simulink model "task2"  (R2025b)
settings: Solver=VariableStepAuto  StartTime=0.0  StopTime=24  RelTol=1e-3
values from neighbouring files (symbols this model uses):
  Pf = 1.5    [init.m]
  Pr = 7.0    (= 7)    [init.m]
  Sb_0 = 0.55    [init.m]
  Ta_0 = 10.0    (= 10)    [init.m]
  Tp_0 = 11.5    [init.m]
libraries: slpidlib x2
settings Model: Creator=davide  LastModifiedBy=davide

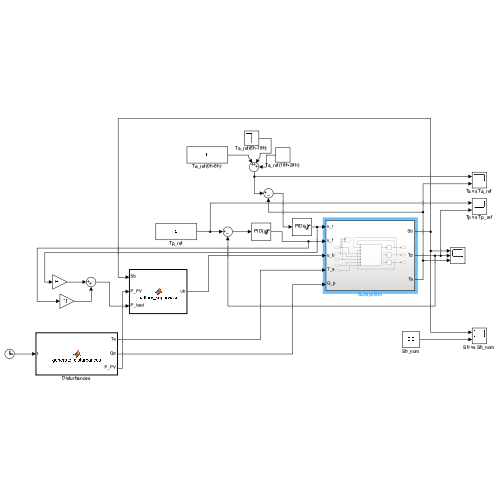
[thumbnail: Simulink's stored preview of the top-level diagram]
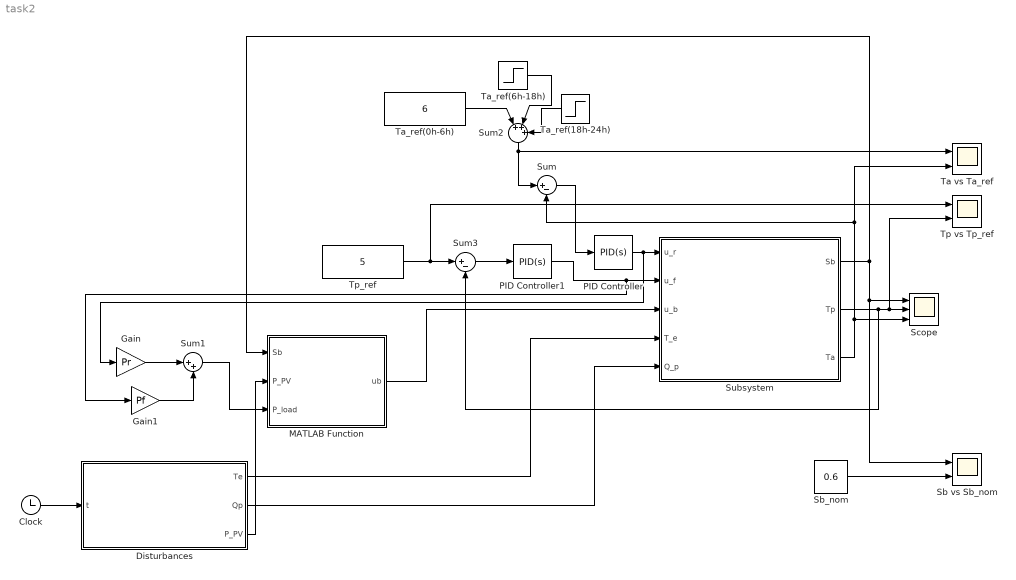
== system task2 ==
  Clock : Clock
  Disturbances : MATLAB Function  TreatAsAtomicUnit=on
  Gain : Gain  Gain=Pr
  Gain1 : Gain  Gain=Pf
  MATLAB Function : MATLAB Function  TreatAsAtomicUnit=on
  PID Controller : slpidlib/PID Controller  Controller=PID  Form=Parallel  TimeDomain=Continuous-time  UseExternalTs=off  SampleTime=-1  IntegratorMethod=Forward Euler  FilterMethod=Forward Euler  ControllerParametersSource=internal  P=-0.5  I=-1  UseKiTs=off  D=0  UseExternalDerivativeSource=off  N=100  UseFilter=on  TunerSelectOption=Transfer Function Based (PID Tuner App)  InitialConditionSource=internal  InitialConditionForIntegrator=0  InitialConditionForFilter=0  DifferentiatorICPrevScaledInput=0  ExternalReset=none  TrackingMode=off  Kt=1  LimitOutput=on  SatLimitsSource=internal  UpperSaturationLimit=1  LowerSaturationLimit=0  LinearizeAsGain=on  AntiWindupMode=back-calculation  Kb=1  LimitIntegrator=off  UpperIntegratorSaturationLimit=inf  LowerIntegratorSaturationLimit=-inf  POutMin=[]  POutMax=[]  IOutMin=[]  IOutMax=[]  DOutMin=[]  DOutMax=[]  NOutMin=[]  NOutMax=[]  SumOutMin=[]  SumOutMax=[]  SaturationOutMin=[]  SaturationOutMax=[]  PParamMin=[]  PParamMax=[]  IParamMin=[]  IParamMax=[]  DParamMin=[]  DParamMax=[]  NParamMin=[]  NParamMax=[]  KbParamMin=[]  KbParamMax=[]  KtParamMin=[]  KtParamMax=[]  KbOutMin=[]  KbOutMax=[]  KtOutMin=[]  KtOutMax=[]  IntegratorOutMin=[]  IntegratorOutMax=[]  FilterOutMin=[]  FilterOutMax=[]  SumI1OutMin=[]  SumI1OutMax=[]  SumI2OutMin=[]  SumI2OutMax=[]  SumI3OutMin=[]  SumI3OutMax=[]  SumI4OutMin=[]  SumI4OutMax=[]  SumDOutMin=[]  SumDOutMax=[]  DifferentiatorOutMin=[]  DifferentiatorOutMax=[]  FilterDiffOutCoefMin=[]  FilterDiffOutCoefMax=[]  ReciprocalOutMin=[]  ReciprocalOutMax=[]  SumDenOutMin=[]  SumDenOutMax=[]  SumNumOutMin=[]  SumNumOutMax=[]  DivideOutMin=[]  DivideOutMax=[]  UdiffTsProdOutMin=[]  UdiffTsProdOutMax=[]  NTsProdOutMin=[]  NTsProdOutMax=[]  UintegralTsProdOutMin=[]  UintegralTsProdOutMax=[]  UngainTsProdOutMin=[]  UngainTsProdOutMax=[]  ClampingZeroOutDataTypeStr=Inherit: Inherit via back propagation  ClampingZeroOutMin=[]  ClampingZeroOutMax=[]  FilterDenConstantOutDataTypeStr=Inherit: Inherit via back propagation  FilterDenConstantOutMin=[]  FilterDenConstantOutMax=[]  PCopyOutDataTypeStr=Inherit: Inherit via back propagation  PCopyOutMin=[]  PCopyOutMax=[]  NCopyOutDataTypeStr=Inherit: Inherit via back propagation  NCopyOutMin=[]  NCopyOutMax=[]  IntegratorContinuousStateAttributes=''  IntegratorStateMustResolveToSignalObject=off  IntegratorRTWStateStorageClass=Auto  FilterContinuousStateAttributes=''  FilterStateMustResolveToSignalObject=off  FilterRTWStateStorageClass=Auto  ParallelPVariant=InternalParameters  IdealPVariant=Disabled  IVariant=InternalParameters  DVariant=InternalParameters  IntegratorVariant=Continuous  SatVariant=Enabled  AWVariant=BackCalculation  PCopyVariant=Disabled  TRVariant=Disabled  FdbkBlocksVariant=Forward  IdealPFdbkVariant=Disabled  SatFdbkVariant=Disabled  DerivativeFilterVariant=ContFilter  NVariant=InternalParameters  NCopyVariant=Disabled  FilterICVariant=InternalICsFilter  IntegratorICVariant=InternalICs  ExternalResetVariant=Disabled  TRSumVariant=Passthrough  SumFdbkVariant=Disabled  SumVariant=Sum_PID  TsampFilterVariant=InternalTs  TsampNgainVariant=Passthrough  TsampIntegralVariant=Disabled_SignalSpec  ExternalSaturationOutDataTypeStr=Inherit: Same as second input  DerivativeSourceVariant=ErrorSignal  PreIntVariant=InternalPreInt
  PID Controller1 : slpidlib/PID Controller  Controller=PID  Form=Parallel  TimeDomain=Continuous-time  UseExternalTs=off  SampleTime=-1  IntegratorMethod=Forward Euler  FilterMethod=Forward Euler  ControllerParametersSource=internal  P=-0.5  I=-1  UseKiTs=off  D=0  UseExternalDerivativeSource=off  N=100  UseFilter=on  TunerSelectOption=Transfer Function Based (PID Tuner App)  InitialConditionSource=internal  InitialConditionForIntegrator=0  InitialConditionForFilter=0  DifferentiatorICPrevScaledInput=0  ExternalReset=none  TrackingMode=off  Kt=1  LimitOutput=on  SatLimitsSource=internal  UpperSaturationLimit=1  LowerSaturationLimit=0  LinearizeAsGain=on  AntiWindupMode=back-calculation  Kb=1  LimitIntegrator=off  UpperIntegratorSaturationLimit=inf  LowerIntegratorSaturationLimit=-inf  POutMin=[]  POutMax=[]  IOutMin=[]  IOutMax=[]  DOutMin=[]  DOutMax=[]  NOutMin=[]  NOutMax=[]  SumOutMin=[]  SumOutMax=[]  SaturationOutMin=[]  SaturationOutMax=[]  PParamMin=[]  PParamMax=[]  IParamMin=[]  IParamMax=[]  DParamMin=[]  DParamMax=[]  NParamMin=[]  NParamMax=[]  KbParamMin=[]  KbParamMax=[]  KtParamMin=[]  KtParamMax=[]  KbOutMin=[]  KbOutMax=[]  KtOutMin=[]  KtOutMax=[]  IntegratorOutMin=[]  IntegratorOutMax=[]  FilterOutMin=[]  FilterOutMax=[]  SumI1OutMin=[]  SumI1OutMax=[]  SumI2OutMin=[]  SumI2OutMax=[]  SumI3OutMin=[]  SumI3OutMax=[]  SumI4OutMin=[]  SumI4OutMax=[]  SumDOutMin=[]  SumDOutMax=[]  DifferentiatorOutMin=[]  DifferentiatorOutMax=[]  FilterDiffOutCoefMin=[]  FilterDiffOutCoefMax=[]  ReciprocalOutMin=[]  ReciprocalOutMax=[]  SumDenOutMin=[]  SumDenOutMax=[]  SumNumOutMin=[]  SumNumOutMax=[]  DivideOutMin=[]  DivideOutMax=[]  UdiffTsProdOutMin=[]  UdiffTsProdOutMax=[]  NTsProdOutMin=[]  NTsProdOutMax=[]  UintegralTsProdOutMin=[]  UintegralTsProdOutMax=[]  UngainTsProdOutMin=[]  UngainTsProdOutMax=[]  ClampingZeroOutDataTypeStr=Inherit: Inherit via back propagation  ClampingZeroOutMin=[]  ClampingZeroOutMax=[]  FilterDenConstantOutDataTypeStr=Inherit: Inherit via back propagation  FilterDenConstantOutMin=[]  FilterDenConstantOutMax=[]  PCopyOutDataTypeStr=Inherit: Inherit via back propagation  PCopyOutMin=[]  PCopyOutMax=[]  NCopyOutDataTypeStr=Inherit: Inherit via back propagation  NCopyOutMin=[]  NCopyOutMax=[]  IntegratorContinuousStateAttributes=''  IntegratorStateMustResolveToSignalObject=off  IntegratorRTWStateStorageClass=Auto  FilterContinuousStateAttributes=''  FilterStateMustResolveToSignalObject=off  FilterRTWStateStorageClass=Auto  ParallelPVariant=InternalParameters  IdealPVariant=Disabled  IVariant=InternalParameters  DVariant=InternalParameters  IntegratorVariant=Continuous  SatVariant=Enabled  AWVariant=BackCalculation  PCopyVariant=Disabled  TRVariant=Disabled  FdbkBlocksVariant=Forward  IdealPFdbkVariant=Disabled  SatFdbkVariant=Disabled  DerivativeFilterVariant=ContFilter  NVariant=InternalParameters  NCopyVariant=Disabled  FilterICVariant=InternalICsFilter  IntegratorICVariant=InternalICs  ExternalResetVariant=Disabled  TRSumVariant=Passthrough  SumFdbkVariant=Disabled  SumVariant=Sum_PID  TsampFilterVariant=InternalTs  TsampNgainVariant=Passthrough  TsampIntegralVariant=Disabled_SignalSpec  ExternalSaturationOutDataTypeStr=Inherit: Same as second input  DerivativeSourceVariant=ErrorSignal  PreIntVariant=InternalPreInt
  Sb vs Sb_nom : Scope  NumInputPorts=2
      settings: ActiveDisplayYMinimum=0.5353840664589169  ActiveDisplayYMaximum=0.65583336699424022  DataLoggingVariableName=ScopeData3
  Sb_nom : Constant  Value=0.6
  Scope : Scope  NumInputPorts=3
      settings: ActiveDisplayYMinimum=-6.671325298198898  ActiveDisplayYMaximum=12.958699337924223
  Subsystem : Subsystem
  Sum : Sum  Inputs=|+-
  Sum1 : Sum  Inputs=|++
  Sum2 : Sum  Inputs=|+++
  Sum3 : Sum  Inputs=|+-
  Ta vs Ta_ref : Scope  NumInputPorts=2
      settings: ActiveDisplayYMinimum=-1  ActiveDisplayYMaximum=1
  Ta_ref(0h-6h) : Constant  Value=6
  Ta_ref(18h-24h) : Step  Time=18  After=-1  SampleTime=0
  Ta_ref(6h-18h) : Step  Time=6  After=-1  SampleTime=0
  Tp vs Tp_ref : Scope  NumInputPorts=2
      settings: ActiveDisplayYMinimum=3.023892907886041  ActiveDisplayYMaximum=12.441789676901552  DataLoggingVariableName=ScopeData2
  Tp_ref : Constant  Value=5
  wires:
  Clock/1 -> Disturbances/1(t)
  Disturbances/1(Te) -> Subsystem/4(T_e)
  Disturbances/2(Qp) -> Subsystem/5(Q_p)
  Subsystem/3(Ta) -> Ta vs Ta_ref/2, Sum/2, Scope/3
  Subsystem/2(Tp) -> Tp vs Tp_ref/2, Scope/2, Sum3/2
  Subsystem/1(Sb) -> Sb vs Sb_nom/1, Scope/1, MATLAB Function/1(Sb)
  Ta_ref(18h-24h)/1 -> Sum2/3
  Ta_ref(6h-18h)/1 -> Sum2/2
  Ta_ref(0h-6h)/1 -> Sum2/1
  Sum2/1 -> Sum/1, Ta vs Ta_ref/1
  Sum/1 -> PID Controller/1
  PID Controller/1 -> Gain/1, Subsystem/1(u_r)
  Tp_ref/1 -> Tp vs Tp_ref/1, Sum3/1
  Sum3/1 -> PID Controller1/1
  PID Controller1/1 -> Gain1/1, Subsystem/2(u_f)
  MATLAB Function/1(ub) -> Subsystem/3(u_b)
  Disturbances/3(P_PV) -> MATLAB Function/2(P_PV)
  Gain1/1 -> Sum1/2
  Gain/1 -> Sum1/1
  Sum1/1 -> MATLAB Function/3(P_load)
  Sb_nom/1 -> Sb vs Sb_nom/2

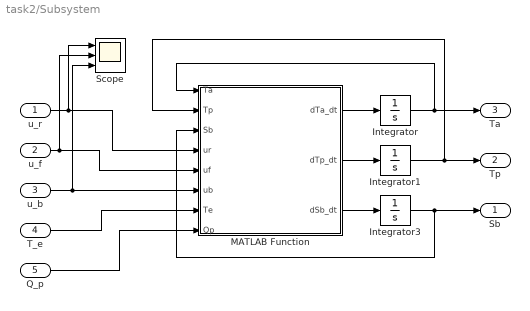
== system task2/Subsystem ==
  u_r : Inport
  u_f : Inport  Port=2
  u_b : Inport  Port=3
  T_e : Inport  Port=4
  Q_p : Inport  Port=5
  Integrator : Integrator  InitialCondition=Ta_0
  Integrator1 : Integrator  InitialCondition=Tp_0
  Integrator3 : Integrator  InitialCondition=Sb_0
  MATLAB Function : MATLAB Function  TreatAsAtomicUnit=on
  Scope : Scope  NumInputPorts=3
      settings: ActiveDisplayYMinimum=-2.5055573579470907  ActiveDisplayYMaximum=4.5560120035571687  DataLoggingVariableName=ScopeData4
  Sb : Outport
  Tp : Outport  Port=2
  Ta : Outport  Port=3
  wires:
  MATLAB Function/1(dTa_dt) -> Integrator/1
  MATLAB Function/2(dTp_dt) -> Integrator1/1
  MATLAB Function/3(dSb_dt) -> Integrator3/1
  Integrator3/1 -> Sb/1, MATLAB Function/3(Sb)
  Integrator/1 -> Ta/1, MATLAB Function/1(Ta)
  Integrator1/1 -> MATLAB Function/2(Tp), Tp/1
  u_r/1 -> MATLAB Function/4(ur), Scope/1
  u_f/1 -> MATLAB Function/5(uf), Scope/2
  u_b/1 -> Scope/3, MATLAB Function/6(ub)
  T_e/1 -> MATLAB Function/7(Te)
  Q_p/1 -> MATLAB Function/8(Qp)

== matlab function task2/Disturbances ==
  data: t input; Te output; Qp output; P_PV output
function [Te, Qp, P_PV] = generate_disturbances(t)
    Rmax = 850; Pmax = 9.0;
    
    Te = 24 + 8 * sin(pi/12 * (t - 8));
    
    if t >= 6 && t <= 18
        Rs = Rmax * sin(pi * (t - 6) / 12);
    else
        Rs = 0;
    end
    P_PV = Pmax * (Rs / Rmax);
    
    % Thermal Charge   
    if t < 4
        Qp = 1200;
    elseif t < 10
        Qp = 600;
    else
        Qp = 250;
    end
end

== matlab function task2/Subsystem/MATLAB Function ==
  data: Ta input; dTa_dt output; Tp input; Sb input; ur input; uf input; ub input; Te input; Qp input; dTp_dt output; dSb_dt output
function [dTa_dt, dTp_dt, dSb_dt] = plant_equations(Ta, Tp, Sb, ur, uf, ub, Te, Qp)
    Ca = 1.5e5; Cp = 8.0e5; ke = 3.8*70; kr = 1.6e4; kf = 450; alpha_f = 1.0;
    Eb = 18; eta_b = 0.94; sec2hour = 3600;

    % Saturations
    ur = max(0, min(1, ur));
    uf = max(0, min(1, uf));
    ub = max(-4, min(4, ub));
    
    if (Sb <= 0.15 && ub < 0) || (Sb >= 0.95 && ub > 0)
        ub = 0; 
    end

    % sec2hour
    dTa_dt = (sec2hour / Ca) * (ke * (Te - Ta) - kr * ur - kf * (1 + alpha_f * uf) * (Ta - Tp) + Qp);
    dTp_dt = (sec2hour / Cp) * (kf * (1 + alpha_f * uf) * (Ta - Tp));
    dSb_dt = (1 / Eb) * ( eta_b * max(-ub, 0) - (1 / eta_b) * max(ub, 0) );
end

== matlab function task2/MATLAB Function ==
  data: Sb input; ub output; P_PV input; P_load input
function ub = battery_supervisor(Sb, P_PV, P_load)
    Sb_nom = 0.60;
    ub_max = 4.0;  % [kW] 
    ub_min = -4.0; % [kW] 
    
    % Calcolo del bilancio netto di potenza
    P_net = P_load - P_PV; 
    
    Kb = 100;

    % Se Sb < Sb_nom, P_soc diventa negativo (richiesta di ricarica)
    P_soc = -Kb * (Sb_nom - Sb); 
    
    % Azione richiesta teorica (Feedforward + Proporzionale)
    ub_req = P_net + P_soc;
    
    
    % Vincolo Bonus: "Battery charging only when surplus PV is available"
    % MASSIMIZZARE la sostenibilità
    if ub_req < 0 
        if P_net >= 0
            % Controlliamo il bilancio energetico reale. Se P_net è positivo, significa che i
            % motori stanno consumando più di quanto il sole produca. In questa situazione, 
            % non c'è energia solare in avanzo. Se caricassimo la batteria, staremmo letteralmente comprando energia dalla rete 
            % per metterla nella batteria, il che è uno spreco economico! Quindi blocchiamo la carica: ub_req = 0
            ub_req = 0;
        else
            % Surplus disponibile: carica la batteria ma senza superare il surplus stesso
            ub_req = max(ub_req, P_net); 
        end
    end
    
    % Limiti di sicurezza dello Stato di Carica (evitiamo i limiti fisici 0.15 e 0.95)
    if Sb <= 0.20 && ub_req > 0
        % Batteria prossima alla scarica critica: ferma l'erogazione
        ub_req = 0; 
    elseif Sb >= 0.90 && ub_req < 0
        % Batteria quasi piena: ferma la ricarica
        ub_req = 0; 
    end
    
    % Saturazione hardware dell'inverter (-4 <= ub <= 4 kW)
    ub = max(ub_min, min(ub_max, ub_req));
end
